simulink model "simulinksim_drive"  (R2025b)
settings: Solver=FixedStepAuto  StartTime=0.0  StopTime=inf  FixedStep=0.001  MaxStep=0.0001  MinStep=0.0001  RelTol=1e-3
model workspace (MAT data in the model file):
  L = 0.57
  La = 0.000279
  Ra = 0.288
  ahead = 0.75
  d = 0.74
  maxrpm = 6000
  pathx : Simulink.Parameter (value not decoded)
  pathy : Simulink.Parameter (value not decoded)
  rover_accel = 0.5
  roveracc = 0.5
  stepangle = 1.8
  w_r = 0.1
  wheelbase = 1
libraries: fl_lib x80, nesl_utility x52, ee_lib x14, slpidlib x6, sdl_lib x6, simulink x4
(part 4 of 4)

== system simulinksim_drive/steppermotorRF/IC Analog Output Vref ==
  SL : Inport
  Controlled Voltage Source : fl_lib/Electrical/Electrical Sources/Controlled Voltage Source
  ERef : fl_lib/Electrical/Electrical Elements/Electrical Reference
  Simulink-PS Converter : nesl_utility/Simulink-PS Converter  PhysicalDomain=network_engine_domain  SubClassName=ps_input  LeftPortType=input  RightPortType=output  PseudoPeriodic=off  Frequencies=[]  NoiseDistribution=none  NoiseParameters=[]  Unit=V  AffineConversion=off  FilteringAndDerivatives=zero  SimscapeFilterOrder=1  InputFilterTimeConstant=.001  UdotUserProvided=0
  V : PMIOPort  Side=Right
  wires:
  SL/1 -> Simulink-PS Converter/1
  connections:
  Simulink-PS Converter/RConn1 -- Controlled Voltage Source/RConn1
  V/RConn1 -- Controlled Voltage Source/LConn1
  ERef/LConn1 -- Controlled Voltage Source/RConn2

== matlab function simulinksim_drive/control_drive/getting the wheel speeds from the turning radii ==
  data: desChassisSpeed input; wheel_speed_LF output; wheel_r input; R input; wheelBase input; R_left input; R_right input; wheel_speed_LM output; wheel_speed_LB output; wheel_speed_RF output; wheel_speed_RM output; wheel_speed_RB output
function [wheel_speed_LF,wheel_speed_LM,wheel_speed_LB,wheel_speed_RF,wheel_speed_RM,wheel_speed_RB] = ...
          ackermann_speeds(desChassisSpeed,wheel_r,R,wheelBase,R_left,R_right)

gearRatio = 10;

if R > 0
    wheel_speed_LF = (desChassisSpeed/wheel_r)*sqrt(R_left^2 + (wheelBase/2)^2)/R;
    wheel_speed_LM = desChassisSpeed * R_left/(R*wheel_r);
    wheel_speed_LB = (desChassisSpeed/wheel_r)*sqrt(R_left^2 + (wheelBase/2)^2)/R;
    wheel_speed_RF = (desChassisSpeed/wheel_r)*sqrt(R_right^2 + (wheelBase/2)^2)/R;
    wheel_speed_RM = desChassisSpeed * R_right/(R*wheel_r);
    wheel_speed_RB = (desChassisSpeed/wheel_r)*sqrt(R_right^2 + (wheelBase/2)^2)/R;
else
    wheel_speed_LF = desChassisSpeed / wheel_r;
    wheel_speed_LM = desChassisSpeed / wheel_r;
    wheel_speed_LB = desChassisSpeed / wheel_r;
    wheel_speed_RF = desChassisSpeed / wheel_r;
    wheel_speed_RM = desChassisSpeed / wheel_r;
    wheel_speed_RB = desChassisSpeed / wheel_r;
end
%{
    wheel_speed_LF = wheel_speed_LF * gearRatio;
    wheel_speed_LM = wheel_speed_LM * gearRatio;
    wheel_speed_LB = wheel_speed_LB * gearRatio;
    wheel_speed_RF = wheel_speed_RF * gearRatio;
    wheel_speed_RM = wheel_speed_RM * gearRatio;
    wheel_speed_RB = wheel_speed_RB * gearRatio;
%}
end

== matlab function simulinksim_drive/control_drive/getting the steering angles and turing radii ==
  data: R input; deltaL output; deltaR output; R output; R_left output; R_right output; wheelBase input; track input
function [deltaL,deltaR,R,R_left,R_right] = ackermann_angles(R,wheelBase,track)
    % Function to compute ackerman steering angles
    if R < 0
        R_left = (R+track/2);
        R_right = (R-track/2);
        deltaL = atan(wheelBase/(R_left));
        deltaR = atan(wheelBase/(R_right));
    elseif R > 0
        R_left = (R-track/2);
        R_right = (R+track/2);
        deltaL = -atan(wheelBase/(R_left));
        deltaR = -atan(wheelBase/(R_right));
    else
        deltaL = 0;
        deltaR = 0;
        R_left = R;
        R_right = R;
    end
    R = abs(R);
end

== matlab function simulinksim_drive/MATLAB Function ==
  data: wheelSpeeds input; wheelRadius input; totalDist output; speed output; deltaTime input
function [totalDist, speed]= chassisSpeed(wheelSpeeds, wheelRadius, deltaTime)
%stays between function calls
persistent distSum

%initialize on first run
if isempty(distSum)
    distSum = 0;
end

wavg = mean(wheelSpeeds);
speed = wavg * wheelRadius;

dist = speed * deltaTime;

distSum = distSum + dist;

%return cumulative distance
totalDist = distSum;

end

== matlab function simulinksim_drive/control_drive/setting the desired speed of the shassis ==
  data: current input; out output; desired input; accelleration input; decelleration input; deltaTime input
function out = linear_interpolation(current, desired, accelleration, decelleration, deltaTime)
%accellerating slower than decellerating
if current >= 0
    if current < desired
        current = current + accelleration * deltaTime;
    end
    if current > desired
        current = current - decelleration * deltaTime;
    end
end
%doing the same going backwards
if current <= 0
    if current > desired
        current = current - accelleration * deltaTime;
    end
    if current < desired
        current = current + decelleration * deltaTime;
    end
end
out = current;
